simulink model "test_compare"  (R2023a)
settings: Solver=FixedStepAuto  StartTime=0.0  StopTime=10.0  FixedStep=0.002  RelTol=1e-3
PreLoadFcn:
  | xt = importrobot('urdf\XT_PRU_noHands.urdf', 'MaxNumBodies', 25);
  | xt.DataFormat = 'col';
  | 
  | urdfPath = "urdf/XT_PRU_noHands.urdf";
libraries: RoboticsCode x100, robotmaniplib x50
(part 2 of 2)

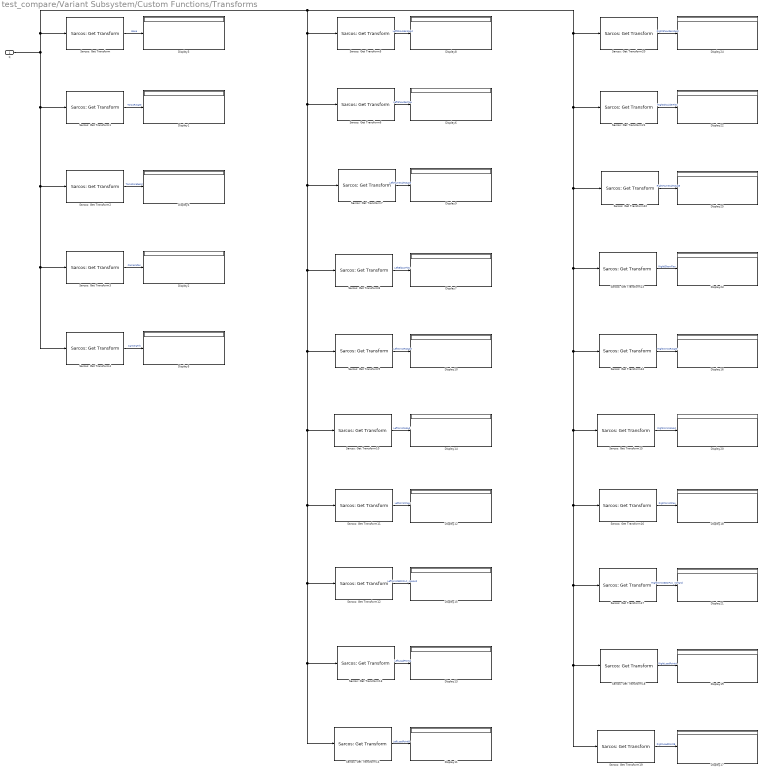
== system test_compare/Variant Subsystem/Custom Functions/Transforms ==
  q : Inport
  Display{1..25} (25 alike) : Display
  Sarcos: Get Transform : RoboticsCode/Sarcos: Get Transform  urdfpath='XT_PRU_noHands.urdf'  source=Base  source_string='Base'  target=World  target_string='World'
      settings: SourceProductName=Sacros Robotics Toolbox
  Sarcos: Get Transform1 : RoboticsCode/Sarcos: Get Transform  urdfpath='XT_PRU_noHands.urdf'  source=TorsoRotate  source_string='TorsoRotate'  target=World  target_string='World'
      settings: SourceProductName=Sacros Robotics Toolbox
  Sarcos: Get Transform10 : RoboticsCode/Sarcos: Get Transform  urdfpath='XT_PRU_noHands.urdf'  source=LeftWristAbAd  source_string='LeftWristAbAd'  target=World  target_string='World'
      settings: SourceProductName=Sacros Robotics Toolbox
  Sarcos: Get Transform11 : RoboticsCode/Sarcos: Get Transform  urdfpath='XT_PRU_noHands.urdf'  source=LeftWristFlex  source_string='LeftWristFlex'  target=World  target_string='World'
      settings: SourceProductName=Sacros Robotics Toolbox
  Sarcos: Get Transform12 : RoboticsCode/Sarcos: Get Transform  urdfpath='XT_PRU_noHands.urdf'  source=LeftWrist6DOFLC_noHand  source_string='LeftWrist6DOFLC_noHand'  target=World  target_string='World'
      settings: SourceProductName=Sacros Robotics Toolbox
  Sarcos: Get Transform13 : RoboticsCode/Sarcos: Get Transform  urdfpath='XT_PRU_noHands.urdf'  source=LeftLoadPointA  source_string='LeftLoadPointA'  target=World  target_string='World'
      settings: SourceProductName=Sacros Robotics Toolbox
  Sarcos: Get Transform14 : RoboticsCode/Sarcos: Get Transform  urdfpath='XT_PRU_noHands.urdf'  source=LeftLoadPointB  source_string='LeftLoadPointB'  target=World  target_string='World'
      settings: SourceProductName=Sacros Robotics Toolbox
  Sarcos: Get Transform15 : RoboticsCode/Sarcos: Get Transform  urdfpath='XT_PRU_noHands.urdf'  source=RightWristAbAd  source_string='RightWristAbAd'  target=World  target_string='World'
      settings: SourceProductName=Sacros Robotics Toolbox
  Sarcos: Get Transform16 : RoboticsCode/Sarcos: Get Transform  urdfpath='XT_PRU_noHands.urdf'  source=RightWristFlex  source_string='RightWristFlex'  target=World  target_string='World'
      settings: SourceProductName=Sacros Robotics Toolbox
  Sarcos: Get Transform17 : RoboticsCode/Sarcos: Get Transform  urdfpath='XT_PRU_noHands.urdf'  source=RightWrist6DOFLC_noHand  source_string='RightWrist6DOFLC_noHand'  target=World  target_string='World'
      settings: SourceProductName=Sacros Robotics Toolbox
  Sarcos: Get Transform18 : RoboticsCode/Sarcos: Get Transform  urdfpath='XT_PRU_noHands.urdf'  source=RightLoadPointA  source_string='RightLoadPointA'  target=World  target_string='World'
      settings: SourceProductName=Sacros Robotics Toolbox
  Sarcos: Get Transform19 : RoboticsCode/Sarcos: Get Transform  urdfpath='XT_PRU_noHands.urdf'  source=RightLoadPointB  source_string='RightLoadPointB'  target=World  target_string='World'
      settings: SourceProductName=Sacros Robotics Toolbox
  Sarcos: Get Transform2 : RoboticsCode/Sarcos: Get Transform  urdfpath='XT_PRU_noHands.urdf'  source=TorsoForebend  source_string='TorsoForebend'  target=World  target_string='World'
      settings: SourceProductName=Sacros Robotics Toolbox
  Sarcos: Get Transform20 : RoboticsCode/Sarcos: Get Transform  urdfpath='XT_PRU_noHands.urdf'  source=RightShoulderAbAd  source_string='RightShoulderAbAd'  target=World  target_string='World'
      settings: SourceProductName=Sacros Robotics Toolbox
  Sarcos: Get Transform21 : RoboticsCode/Sarcos: Get Transform  urdfpath='XT_PRU_noHands.urdf'  source=RightShoulderFlex  source_string='RightShoulderFlex'  target=World  target_string='World'
      settings: SourceProductName=Sacros Robotics Toolbox
  Sarcos: Get Transform22 : RoboticsCode/Sarcos: Get Transform  urdfpath='XT_PRU_noHands.urdf'  source=RightHumeralRotate  source_string='RightHumeralRotate'  target=World  target_string='World'
      settings: SourceProductName=Sacros Robotics Toolbox
  Sarcos: Get Transform23 : RoboticsCode/Sarcos: Get Transform  urdfpath='XT_PRU_noHands.urdf'  source=RightElbowFlex  source_string='RightElbowFlex'  target=World  target_string='World'
      settings: SourceProductName=Sacros Robotics Toolbox
  Sarcos: Get Transform24 : RoboticsCode/Sarcos: Get Transform  urdfpath='XT_PRU_noHands.urdf'  source=RightWristRotate  source_string='RightWristRotate'  target=World  target_string='World'
      settings: SourceProductName=Sacros Robotics Toolbox
  Sarcos: Get Transform3 : RoboticsCode/Sarcos: Get Transform  urdfpath='XT_PRU_noHands.urdf'  source=CameraPan  source_string='CameraPan'  target=World  target_string='World'
      settings: SourceProductName=Sacros Robotics Toolbox
  Sarcos: Get Transform4 : RoboticsCode/Sarcos: Get Transform  urdfpath='XT_PRU_noHands.urdf'  source=CameraTilt  source_string='CameraTilt'  target=World  target_string='World'
      settings: SourceProductName=Sacros Robotics Toolbox
  Sarcos: Get Transform5 : RoboticsCode/Sarcos: Get Transform  urdfpath='XT_PRU_noHands.urdf'  source=LeftShoulderAbAd  source_string='LeftShoulderAbAd'  target=World  target_string='World'
      settings: SourceProductName=Sacros Robotics Toolbox
  Sarcos: Get Transform6 : RoboticsCode/Sarcos: Get Transform  urdfpath='XT_PRU_noHands.urdf'  source=LeftShoulderFlex  source_string='LeftShoulderFlex'  target=World  target_string='World'
      settings: SourceProductName=Sacros Robotics Toolbox
  Sarcos: Get Transform7 : RoboticsCode/Sarcos: Get Transform  urdfpath='XT_PRU_noHands.urdf'  source=LeftHumeralRotate  source_string='LeftHumeralRotate'  target=World  target_string='World'
      settings: SourceProductName=Sacros Robotics Toolbox
  Sarcos: Get Transform8 : RoboticsCode/Sarcos: Get Transform  urdfpath='XT_PRU_noHands.urdf'  source=LeftElbowFlex  source_string='LeftElbowFlex'  target=World  target_string='World'
      settings: SourceProductName=Sacros Robotics Toolbox
  Sarcos: Get Transform9 : RoboticsCode/Sarcos: Get Transform  urdfpath='XT_PRU_noHands.urdf'  source=LeftWristRotate  source_string='LeftWristRotate'  target=World  target_string='World'
      settings: SourceProductName=Sacros Robotics Toolbox
  wires:
  q/1 -> Sarcos: Get Transform23/1, Sarcos: Get Transform19/1, Sarcos: Get Transform18/1, Sarcos: Get Transform17/1, Sarcos: Get Transform16/1, Sarcos: Get Transform15/1, Sarcos: Get Transform24/1, Sarcos: Get Transform22/1, Sarcos: Get Transform21/1, Sarcos: Get Transform20/1, Sarcos: Get Transform6/1, Sarcos: Get Transform13/1, Sarcos: Get Transform14/1, Sarcos: Get Transform12/1, Sarcos: Get Transform11/1, Sarcos: Get Transform10/1, Sarcos: Get Transform9/1, Sarcos: Get Transform8/1, Sarcos: Get Transform7/1, Sarcos: Get Transform5/1, Sarcos: Get Transform/1, Sarcos: Get Transform2/1, Sarcos: Get Transform3/1, Sarcos: Get Transform4/1, Sarcos: Get Transform1/1
  Sarcos: Get Transform/1 -> Display3/1  "Base"
  Sarcos: Get Transform1/1 -> Display1/1  "TorsoRotate"
  Sarcos: Get Transform2/1 -> Display4/1  "TorsoForebend"
  Sarcos: Get Transform3/1 -> Display2/1  "CameraPan"
  Sarcos: Get Transform4/1 -> Display5/1  "CameraTilt"
  Sarcos: Get Transform5/1 -> Display8/1  "LeftShoulderAbAd"
  Sarcos: Get Transform6/1 -> Display6/1  "LeftShoulderFlex"
  Sarcos: Get Transform7/1 -> Display9/1  "LeftHumeralRotate"
  Sarcos: Get Transform8/1 -> Display7/1  "LeftElbowFlex"
  Sarcos: Get Transform9/1 -> Display10/1  "LeftWristRotate"
  Sarcos: Get Transform10/1 -> Display14/1  "LeftWristAbAd"
  Sarcos: Get Transform11/1 -> Display12/1  "LeftWristFlex"
  Sarcos: Get Transform12/1 -> Display15/1  "LeftWrist6DOFLC_noHand"
  Sarcos: Get Transform13/1 -> Display13/1  "LeftLoadPointA"
  Sarcos: Get Transform14/1 -> Display11/1  "LeftLoadPointB"
  Sarcos: Get Transform20/1 -> Display24/1  "RightShoulderAbAd"
  Sarcos: Get Transform21/1 -> Display22/1  "RightShoulderFlex"
  Sarcos: Get Transform22/1 -> Display25/1  "RightHumeralRotate"
  Sarcos: Get Transform23/1 -> Display23/1  "RightElbowFlex"
  Sarcos: Get Transform24/1 -> Display16/1  "RightWristRotate"
  Sarcos: Get Transform15/1 -> Display20/1  "RightWristAbAd"
  Sarcos: Get Transform16/1 -> Display18/1  "RightWristFlex"
  Sarcos: Get Transform17/1 -> Display21/1  "RightWrist6DOFLC_noHand"
  Sarcos: Get Transform18/1 -> Display19/1  "RightLoadPointA"
  Sarcos: Get Transform19/1 -> Display17/1  "RightLoadPointB"
